simulink model "simu_21a"  (R2021a)
settings: Solver=ode4  StartTime=0.0  StopTime=15  FixedStep=0.01  RelTol=1e-3
libraries: simulink x4, simulink_extras x4
settings Model: Creator=psp_dada  LastModifiedBy=psp_dada
settings DebuggingCC: UnconnectedInputMsg=none  UnconnectedOutputMsg=none  UnconnectedLineMsg=none
settings ModelReferenceCC: EnableRefExpFcnMdlSchedulingChecks=off
settings RTWCC: Description=Generic Real-Time Target  GPUComputeCapability=5.0  DLArmComputeVersion=20.02.1
settings ConfigComp: CovBoundaryAbsTol=1.0e-5

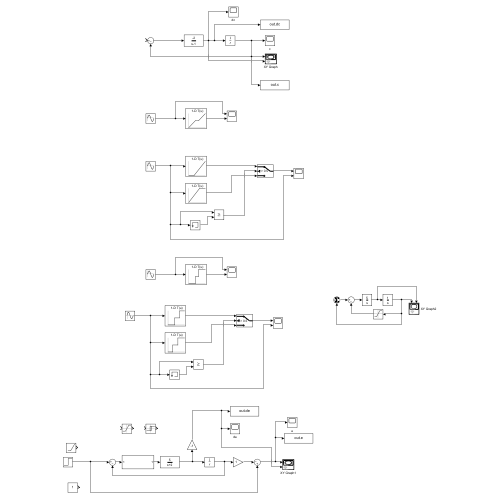
[thumbnail: Simulink's stored preview of the top-level diagram]
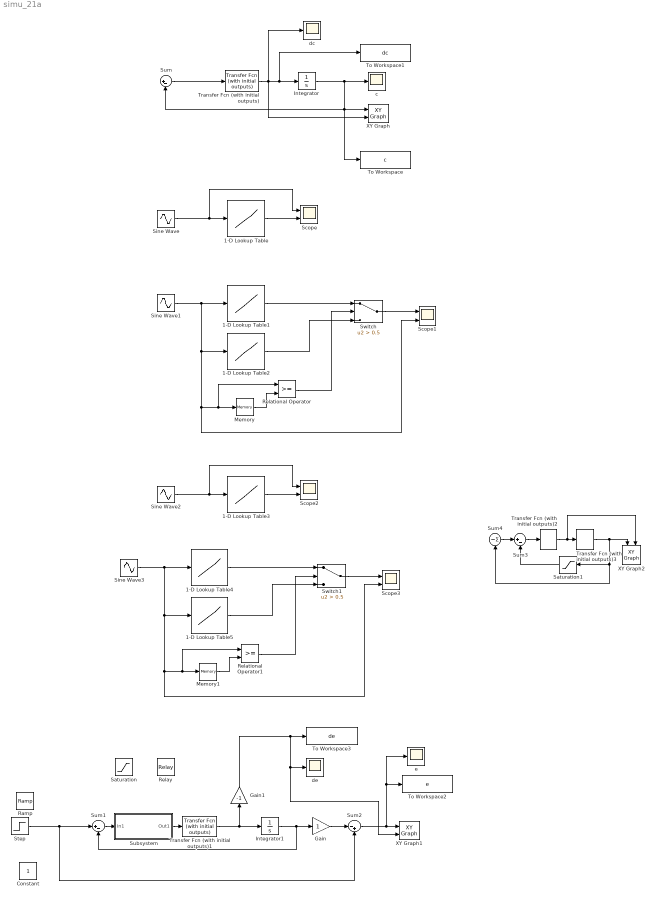
== system simu_21a ==
  1-D Lookup Table : Lookup_n-D  NumberOfTableDimensions=1  BreakpointsForDimension1=[-5 -1 1 5]  Table=[-4 0 0 4]  InternalRulePriority=Speed  RndMeth=Simplest  InputSameDT=on
  1-D Lookup Table1 : Lookup_n-D  NumberOfTableDimensions=1  BreakpointsForDimension1=[-3 -1 3]  Table=[-1 -1 1]  InternalRulePriority=Speed  RndMeth=Simplest  InputSameDT=on
  1-D Lookup Table2 : Lookup_n-D  NumberOfTableDimensions=1  BreakpointsForDimension1=[-3 1 3]  Table=[-1 1 1]  InternalRulePriority=Speed  RndMeth=Simplest  InputSameDT=on
  1-D Lookup Table3 : Lookup_n-D  NumberOfTableDimensions=1  BreakpointsForDimension1=[-5 -1.001 -1 1 1.001 5]  Table=[-1 -1 0 0 1 1]  InternalRulePriority=Speed  RndMeth=Simplest  InputSameDT=on
  1-D Lookup Table4 : Lookup_n-D  NumberOfTableDimensions=1  BreakpointsForDimension1=[-5 -1.001 -1 2 2.001 5]  Table=[-1 -1 0 0 1 1]  InternalRulePriority=Speed  RndMeth=Simplest  InputSameDT=on
  1-D Lookup Table5 : Lookup_n-D  NumberOfTableDimensions=1  BreakpointsForDimension1=[-5 -2.0001 -2 1 1.001 5]  Table=[-1 -1 0 0 1 1]  InternalRulePriority=Speed  RndMeth=Simplest  InputSameDT=on
  Constant : Constant
  Gain : Gain
  Gain1 : Gain  Gain=-1
  Integrator : Integrator  InitialCondition=10
  Integrator1 : Integrator  InitialCondition=-0.5
  Memory : Memory
  Memory1 : Memory
  Ramp : simulink/Sources/Ramp  slope=1  start=0  InitialOutput=0
  Relational Operator : RelationalOperator  OutDataTypeStr=boolean  RndMeth=Simplest
  Relational Operator1 : RelationalOperator  OutDataTypeStr=boolean  RndMeth=Simplest
  Relay : Relay  OnSwitchValue=1  OffSwitchValue=-1  OffOutputValue=-1
  Saturation : Saturate
  Saturation1 : Saturate  UpperLimit=1  LowerLimit=-1
  Scope{,1..3} (4 alike) : Scope  NumInputPorts=2
  Sine Wave : Sin  Amplitude=2  SampleTime=0
  Sine Wave1 : Sin  Amplitude=3  SampleTime=0
  Sine Wave2 : Sin  Amplitude=2  SampleTime=0
  Sine Wave3 : Sin  Amplitude=2  SampleTime=0
  Step : Step  Time=0  After=0  SampleTime=0
  Subsystem : Subsystem
  Sum : Sum  Inputs=|+-
  Sum1 : Sum  Inputs=|+-
  Sum2 : Sum  Inputs=|-+
  Sum3 : Sum  Inputs=|+-
  Sum4 : Sum  Inputs=||-
  Switch : Switch  Criteria=u2 > Threshold  Threshold=0.5
  Switch1 : Switch  Criteria=u2 > Threshold  Threshold=0.5
  To Workspace : ToWorkspace  VariableName=c  SampleTime=-1
  To Workspace1 : ToWorkspace  VariableName=dc  SampleTime=-1
  To Workspace2 : ToWorkspace  VariableName=e  SampleTime=-1
  To Workspace3 : ToWorkspace  VariableName=de  SampleTime=-1
  Transfer Fcn (with initial outputs) : simulink_extras/Additional Linear/Transfer Fcn (with initial outputs)  N=[-2]  D=[1 -1]  Y0=-10.5  U0=0
  Transfer Fcn (with initial outputs)1 : simulink_extras/Additional Linear/Transfer Fcn (with initial outputs)  N=[5]  D=[1 2]  Y0=0.3  U0=0
  Transfer Fcn (with initial outputs)2 : simulink_extras/Additional Linear/Transfer Fcn (with initial outputs)  N=[5]  D=[1 0]  Y0=2  U0=0
  Transfer Fcn (with initial outputs)3 : simulink_extras/Additional Linear/Transfer Fcn (with initial outputs)  N=[1]  D=[1 0]  Y0=2  U0=0
  XY Graph : simulink/Sinks/XY Graph  xmin=-1  xmax=1  ymin=-1  ymax=1  st=-1
  XY Graph1 : simulink/Sinks/XY Graph  xmin=-1  xmax=1  ymin=-1  ymax=1  st=-1
  XY Graph2 : simulink/Sinks/XY Graph  xmin=-1  xmax=1  ymin=-1  ymax=1  st=-1
  c : Scope
  dc : Scope
  de : Scope
  e : Scope
  wires:
  Sum/1 -> Transfer Fcn (with initial outputs)/1
  Transfer Fcn (with initial outputs)/1 -> dc/1, XY Graph/2, To Workspace1/1, Integrator/1
  Integrator/1 -> Sum/2, To Workspace/1, XY Graph/1, c/1
  Sine Wave/1 -> 1-D Lookup Table/1, Scope/1
  1-D Lookup Table/1 -> Scope/2
  Sine Wave1/1 -> 1-D Lookup Table2/1, Relational Operator/1, Memory/1, Scope1/2, 1-D Lookup Table1/1
  1-D Lookup Table1/1 -> Switch/1
  Switch/1 -> Scope1/1
  1-D Lookup Table2/1 -> Switch/3
  Relational Operator/1 -> Switch/2
  Memory/1 -> Relational Operator/2
  Sine Wave2/1 -> 1-D Lookup Table3/1, Scope2/1
  1-D Lookup Table3/1 -> Scope2/2
  Sine Wave3/1 -> 1-D Lookup Table5/1, Relational Operator1/1, Memory1/1, Scope3/2, 1-D Lookup Table4/1
  1-D Lookup Table5/1 -> Switch1/3
  1-D Lookup Table4/1 -> Switch1/1
  Relational Operator1/1 -> Switch1/2
  Switch1/1 -> Scope3/1
  Memory1/1 -> Relational Operator1/2
  Step/1 -> Sum2/2, Sum1/1
  Sum1/1 -> Subsystem/1(In1)
  Subsystem/1(Out1) -> Transfer Fcn (with initial outputs)1/1
  Transfer Fcn (with initial outputs)1/1 -> Integrator1/1, Gain1/1
  Integrator1/1 -> Sum1/2, Gain/1
  Gain1/1 -> XY Graph1/2, de/1, To Workspace3/1
  Gain/1 -> Sum2/1
  Sum2/1 -> To Workspace2/1, e/1, XY Graph1/1
  Saturation1/1 -> Sum3/2
  Sum4/1 -> Sum3/1
  Transfer Fcn (with initial outputs)3/1 -> XY Graph2/1, Sum4/1, Saturation1/1
  Transfer Fcn (with initial outputs)2/1 -> Transfer Fcn (with initial outputs)3/1, XY Graph2/2
  Sum3/1 -> Transfer Fcn (with initial outputs)2/1

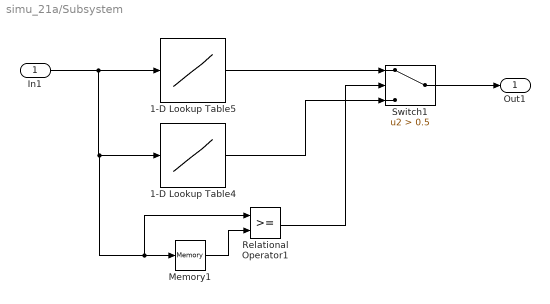
== system simu_21a/Subsystem ==
  In1 : Inport
  1-D Lookup Table4 : Lookup_n-D  NumberOfTableDimensions=1  BreakpointsForDimension1=[-2 -1.001 -1 2]  Table="[-1 -1  1 1]"  InternalRulePriority=Speed  RndMeth=Simplest  InputSameDT=on
  1-D Lookup Table5 : Lookup_n-D  NumberOfTableDimensions=1  BreakpointsForDimension1=[-2 1 1.001 2]  Table=[-1 -1 1 1]  InternalRulePriority=Speed  RndMeth=Simplest  InputSameDT=on
  Memory1 : Memory
  Relational Operator1 : RelationalOperator  OutDataTypeStr=boolean  RndMeth=Simplest
  Switch1 : Switch  Criteria=u2 > Threshold  Threshold=0.5
  Out1 : Outport
  wires:
  In1/1 -> 1-D Lookup Table5/1, 1-D Lookup Table4/1, Relational Operator1/1, Memory1/1
  Memory1/1 -> Relational Operator1/2
  1-D Lookup Table5/1 -> Switch1/1
  Relational Operator1/1 -> Switch1/2
  Switch1/1 -> Out1/1
  1-D Lookup Table4/1 -> Switch1/3
